simulink model "quadrotor_model50"  (R2021a)
settings: Solver=VariableStepAuto  StartTime=0.0  StopTime=40  RelTol=1e-1
values from neighbouring files (symbols this model uses):
  X = [X realx(index)]    [Plot_drone_3D.m]    (also in Plot_drone_3D_sub.m)
  Y = [Y realy(index)]    [Plot_drone_3D.m]    (also in Plot_drone_3D_sub.m)
  Z = [Z realz(index)]    [Plot_drone_3D.m]    (also in Plot_drone_3D_sub.m)
undefined symbols (not defined in the file or in its folder): Discrete, Time
libraries: sm_lib x6, sharedTrackingLibrary x4, sharedtransform x3, vrlib x2, aerolibutil x2, nesl_utility x1, dspmtrx3 x1, ctrlSharedLib x1
(part 2 of 2)

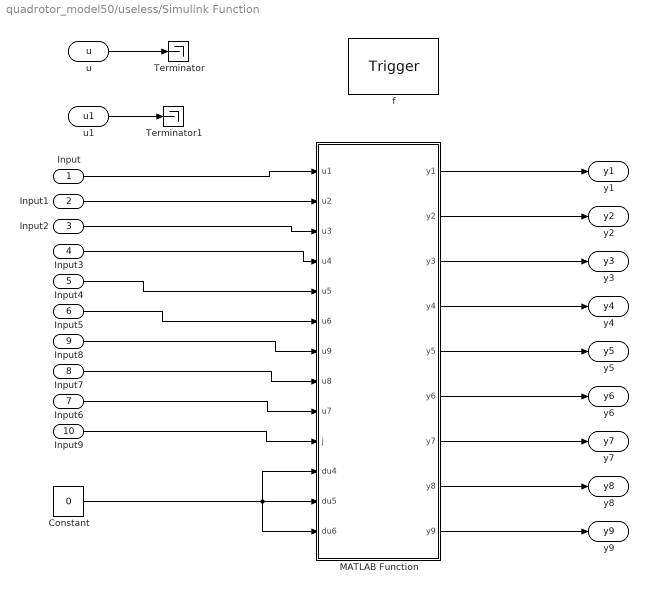
== system quadrotor_model50/useless/Simulink Function ==
  Input : Inport
  Input1 : Inport  Port=2
  Input2 : Inport  Port=3
  Input3 : Inport  Port=4
  Input4 : Inport  Port=5
  Input5 : Inport  Port=6
  Input6 : Inport  Port=7
  Input7 : Inport  Port=8
  Input8 : Inport  Port=9
  Input9 : Inport  Port=10
  f : TriggerPort  TriggerType=function-call  IsSimulinkFunction=on  FunctionName=suktee  FunctionVisibility=scoped  VariantControl=(inherit)
  Constant : Constant  Value=0
  MATLAB Function : MATLAB Function  TreatAsAtomicUnit=on
  Terminator : Terminator
  Terminator1 : Terminator
  u : ArgIn  DisableCoverage=on  ArgumentName=u
  u1 : ArgIn  DisableCoverage=on  Port=2  ArgumentName=u1
  y1 : ArgOut  DisableCoverage=on  ArgumentName=y1
  y2 : ArgOut  DisableCoverage=on  Port=2  ArgumentName=y2
  y3 : ArgOut  DisableCoverage=on  Port=3  ArgumentName=y3
  y4 : ArgOut  DisableCoverage=on  Port=4  ArgumentName=y4
  y5 : ArgOut  DisableCoverage=on  Port=5  ArgumentName=y5
  y6 : ArgOut  DisableCoverage=on  Port=6  ArgumentName=y6
  y7 : ArgOut  DisableCoverage=on  Port=7  ArgumentName=y7
  y8 : ArgOut  DisableCoverage=on  Port=8  ArgumentName=y8
  y9 : ArgOut  DisableCoverage=on  Port=9  ArgumentName=y9
  wires:
  Input/1 -> MATLAB Function/1(u1)
  Input1/1 -> MATLAB Function/2(u2)
  Input2/1 -> MATLAB Function/3(u3)
  Input4/1 -> MATLAB Function/5(u5)
  Input5/1 -> MATLAB Function/6(u6)
  Input7/1 -> MATLAB Function/8(u8)
  Input8/1 -> MATLAB Function/7(u9)
  Input6/1 -> MATLAB Function/9(u7)
  Input9/1 -> MATLAB Function/10(j)
  Input3/1 -> MATLAB Function/4(u4)
  MATLAB Function/1(y1) -> y1/1
  MATLAB Function/2(y2) -> y2/1
  MATLAB Function/3(y3) -> y3/1
  MATLAB Function/4(y4) -> y4/1
  MATLAB Function/5(y5) -> y5/1
  MATLAB Function/6(y6) -> y6/1
  MATLAB Function/9(y9) -> y9/1
  MATLAB Function/8(y8) -> y8/1
  MATLAB Function/7(y7) -> y7/1
  Constant/1 -> MATLAB Function/11(du4), MATLAB Function/13(du6), MATLAB Function/12(du5)
  u/1 -> Terminator/1
  u1/1 -> Terminator1/1

== system quadrotor_model50/useless/Simulink Function1 ==
  Input : Inport
  Input1 : Inport  Port=2
  Input2 : Inport  Port=3
  f : TriggerPort  TriggerType=function-call  IsSimulinkFunction=on  FunctionName=meas  FunctionVisibility=scoped  VariantControl=(inherit)
  y1 : ArgOut  DisableCoverage=on  ArgumentName=y1
  y2 : ArgOut  DisableCoverage=on  Port=2  ArgumentName=y2
  y3 : ArgOut  DisableCoverage=on  Port=3  ArgumentName=y3
  wires:
  Input/1 -> y1/1
  Input1/1 -> y2/1
  Input2/1 -> y3/1

== system quadrotor_model50/useless/Simulink Function2 ==
  jx : Inport
  jy : Inport  Port=2
  jz : Inport  Port=3
  jaba : TriggerPort  TriggerType=function-call  IsSimulinkFunction=on  FunctionName=jaba  FunctionVisibility=scoped  VariantControl=(inherit)
  MATLAB Function4 : MATLAB Function  TreatAsAtomicUnit=on
  y : ArgOut  DisableCoverage=on  ArgumentName=y
  wires:
  jy/1 -> MATLAB Function4/2(jy)
  jx/1 -> MATLAB Function4/1(jx)
  jz/1 -> MATLAB Function4/3(jz)
  MATLAB Function4/1(a) -> y/1

== system quadrotor_model50/useless/Simulink Function3 ==
  Input : Inport
  messi : TriggerPort  TriggerType=function-call  IsSimulinkFunction=on  FunctionName=messi  FunctionVisibility=scoped  VariantControl=(inherit)
  Demux : Demux  Outputs=3
  y : ArgOut  DisableCoverage=on  ArgumentName=y
  y1 : ArgOut  DisableCoverage=on  Port=2  ArgumentName=y1
  y2 : ArgOut  DisableCoverage=on  Port=3  ArgumentName=y2
  wires:
  Demux/3 -> y2/1
  Demux/1 -> y/1
  Demux/2 -> y1/1
  Input/1 -> Demux/1

== system quadrotor_model50/Quadrotor/Dynamics Model/Orientation Dynamics ==
  tau : Inport
  w : Inport  Port=2
  Body Inertia Matrix : Constant  Value=I
  Cross Product : vrlib/Utilities/Cross Product
  Matrix Multiply : Product  Multiplication=Matrix(*)
  Product : Product  Inputs=/*  Multiplication=Matrix(*)  OutDataTypeStr=Inherit: Inherit via back propagation
  Sum : Sum  Inputs=+-|
  dw : Outport
  wires:
  Body Inertia Matrix/1 -> Product/1, Matrix Multiply/1
  Matrix Multiply/1 -> Cross Product/2
  w/1 -> Cross Product/1, Matrix Multiply/2
  Cross Product/1 -> Sum/2
  tau/1 -> Sum/1
  Sum/1 -> Product/2
  Product/1 -> dw/1

== system quadrotor_model50/Quadrotor/Dynamics Model/Position Dynamics ==
  f : Inport
  Mass : Constant  Value=m
  Product1 : Product  Inputs=*/
  dv : Outport
  wires:
  Product1/1 -> dv/1
  f/1 -> Product1/1
  Mass/1 -> Product1/2

== system quadrotor_model50/Quadrotor/KInematics Model /Orientation Kinematics ==
  w : Inport
  q : Inport  Port=2
  Cross Product : vrlib/Utilities/Cross Product
  Demux : Demux
  Dot Product : DotProduct  InputSameDT=on  OutDataTypeStr=Inherit: Inherit via internal rule
  Gain1 : Gain  Gain=-1
  Mux : Mux  Inputs=3
  Mux1 : Mux  Inputs=2
  Product : Product
  Sum : Sum  Inputs=|++
  dq : Outport
  wires:
  q/1 -> Demux/1  "q"
  Demux/2 -> Mux/1
  Demux/3 -> Mux/2
  w/1 -> Product/2, Dot Product/2, Cross Product/2  "w"
  Demux/4 -> Mux/3
  Mux/1 -> Dot Product/1, Cross Product/1  "q_v"
  Mux1/1 -> dq/1
  Demux/1 -> Product/1  "q_0"
  Product/1 -> Sum/1
  Cross Product/1 -> Sum/2
  Sum/1 -> Mux1/2
  Dot Product/1 -> Gain1/1
  Gain1/1 -> Mux1/1

== system quadrotor_model50/Quadrotor/KInematics Model /Position Kinematics ==
  v : Inport
  dp : Outport
  wires:
  v/1 -> dp/1

== system quadrotor_model50/Quadrotor/KInematics Model /Vector Normalization ==
  v : Inport
  Dot Product1 : DotProduct  InputSameDT=on  OutDataTypeStr=Inherit: Inherit via internal rule
  Product3 : Product  Inputs=*/
  Sqrt : Sqrt  SaturateOnIntegerOverflow=on
  v' : Outport
  wires:
  Product3/1 -> v'/1
  v/1 -> Dot Product1/2, Product3/1, Dot Product1/1
  Dot Product1/1 -> Sqrt/1
  Sqrt/1 -> Product3/2

== system quadrotor_model50/Quadrotor/quat2Rotm/Skew Operator ==
  v : Inport
  Constant : Constant  Value=0
  Demux1 : Demux  Outputs=3
  Demux2 : Demux  Outputs=3
  Gain1 : Gain  Gain=-1
  Matrix Concatenate : Concatenate  NumInputs=3  Mode=Multidimensional array  ConcatenateDimension=2
  Mux1 : Mux  Inputs=3
  Mux2 : Mux  Inputs=3
  Mux3 : Mux  Inputs=3
  S : Outport
  wires:
  Constant/1 -> Mux3/3, Mux2/2, Mux1/1
  Demux1/3 -> Mux1/2
  Matrix Concatenate/1 -> S/1
  Demux1/1 -> Mux2/3
  v/1 -> Demux1/1, Gain1/1  "v"
  Demux2/1 -> Mux3/2
  Mux3/1 -> Matrix Concatenate/3
  Gain1/1 -> Demux2/1
  Demux2/3 -> Mux2/1
  Mux1/1 -> Matrix Concatenate/1
  Demux2/2 -> Mux1/3
  Demux1/2 -> Mux3/1
  Mux2/1 -> Matrix Concatenate/2

== system quadrotor_model50/Subsystem1/Subsystem/c ==
  y : Inport  SampleTime=1/100
  In2 : Inport  Port=2
  In3 : Inport  Port=3
  Constant : Constant
  Constant1 : Constant  Value=0
  Cos : Trigonometry  Operator=cos
  Cos1 : Trigonometry  Operator=cos
  Divide : Product  Inputs=**
  Divide1 : Product  Inputs=*/
  MATLAB Function : MATLAB Function  TreatAsAtomicUnit=on
  Mux : Mux  Inputs=36
  Reshape : Reshape  OutputDimensionality=Customize  OutputDimensions=[4,9]
  c : Outport  SampleTime=1/100
  wires:
  In2/1 -> Cos/1
  In3/1 -> Cos1/1
  Cos/1 -> Divide/1
  Cos1/1 -> Divide/2
  Constant/1 -> Divide1/1
  Divide/1 -> Divide1/2
  y/1 -> MATLAB Function/1(u)
  Divide1/1 -> Mux/12
  MATLAB Function/1(r1) -> Mux/25
  MATLAB Function/2(r2) -> Mux/26
  MATLAB Function/3(r3) -> Mux/27
  MATLAB Function/4(r4) -> Mux/29
  MATLAB Function/5(r5) -> Mux/30
  MATLAB Function/6(r6) -> Mux/31
  MATLAB Function/7(r7) -> Mux/33
  MATLAB Function/8(r8) -> Mux/34
  MATLAB Function/9(r9) -> Mux/35
  Constant1/1 -> Mux/24, Mux/23, Mux/22, Mux/21, Mux/20, Mux/19, Mux/18, Mux/17, Mux/16, Mux/15, Mux/14, Mux/13, Mux/11, Mux/10, Mux/9, Mux/8, Mux/7, Mux/6, Mux/5, Mux/4, Mux/3, Mux/2, Mux/1, Mux/28, Mux/32, Mux/36
  Mux/1 -> Reshape/1
  Reshape/1 -> c/1

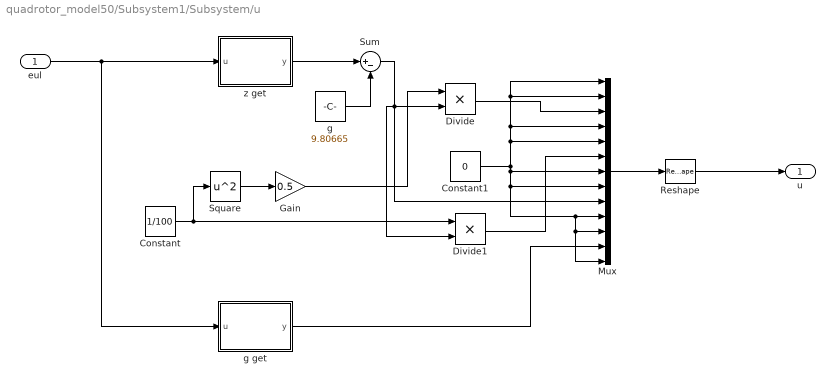
== system quadrotor_model50/Subsystem1/Subsystem/u ==
  eul : Inport
  Constant : Constant  Value=1/100
  Constant1 : Constant  Value=0
  Divide : Product  Inputs=**
  Divide1 : Product  Inputs=**
  Gain : Gain  Gain=0.5
  Mux : Mux  Inputs=13
  Reshape : Reshape  OutputDimensionality=Customize  OutputDimensions=[13,1]
  Square : Math  Operator=square  SaturateOnIntegerOverflow=on
  Sum : Sum  Inputs=|+-
  g : Constant  Value=9.80665
  g get : MATLAB Function  TreatAsAtomicUnit=on
  z get : MATLAB Function  TreatAsAtomicUnit=on
  u : Outport  SampleTime=1/100
  wires:
  Constant/1 -> Divide1/1, Square/1
  Square/1 -> Gain/1
  eul/1 -> g get/1(u), z get/1(u)
  z get/1(y) -> Sum/1
  g/1 -> Sum/2
  Gain/1 -> Divide/1
  Sum/1 -> Mux/9, Divide/2, Divide1/2
  Divide/1 -> Mux/3
  Divide1/1 -> Mux/6
  g get/1(y) -> Mux/12
  Constant1/1 -> Mux/13, Mux/11, Mux/10, Mux/8, Mux/7, Mux/5, Mux/4, Mux/1, Mux/2
  Mux/1 -> Reshape/1
  Reshape/1 -> u/1

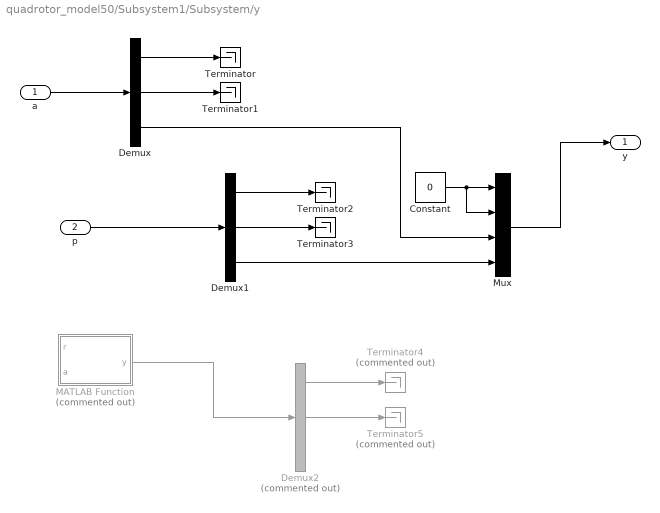
== system quadrotor_model50/Subsystem1/Subsystem/y ==
  a : Inport
  p : Inport  Port=2
  Constant : Constant  Value=0
  Demux : Demux  Outputs=3
  Demux1 : Demux  Outputs=3
  Demux2 : Demux  Commented=on  Outputs=3
  MATLAB Function : MATLAB Function  Commented=on  TreatAsAtomicUnit=on
  Mux : Mux
  Terminator{,1..3} (4 alike) : Terminator
  Terminator4 : Terminator  Commented=on
  Terminator5 : Terminator  Commented=on
  y : Outport  SampleTime=1/100
  wires:
  a/1 -> Demux/1
  Demux/1 -> Terminator/1
  Demux/2 -> Terminator1/1
  Demux1/2 -> Terminator3/1
  p/1 -> Demux1/1
  Demux1/1 -> Terminator2/1
  Demux1/3 -> Mux/4
  Constant/1 -> Mux/2, Mux/1
  Mux/1 -> y/1
  MATLAB Function/1(y) -> Demux2/1
  Demux2/2 -> Terminator5/1
  Demux2/1 -> Terminator4/1
  Demux/3 -> Mux/3

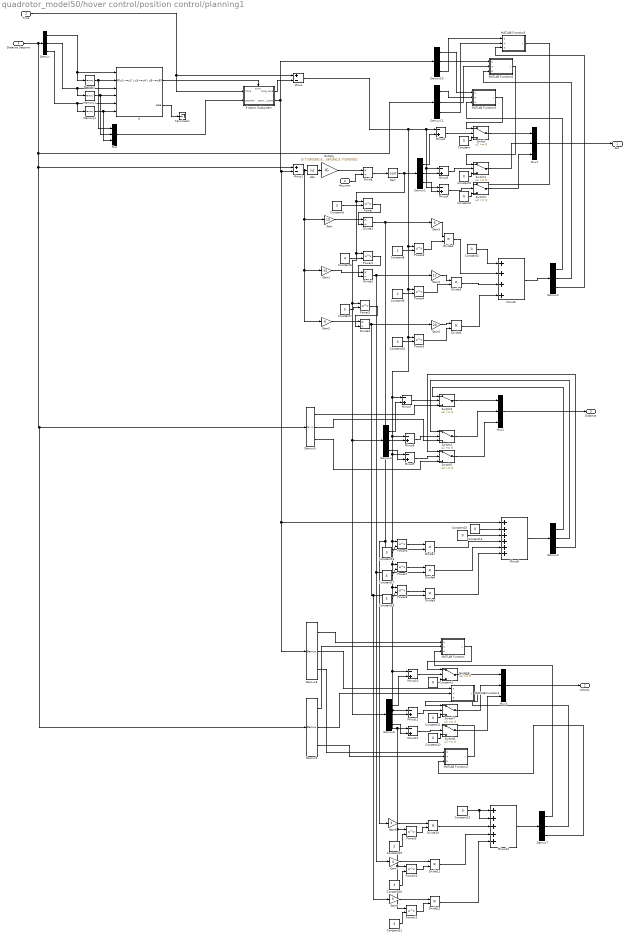
== system quadrotor_model50/hover control/position control/planning1 ==
  Distance Setpoint : Inport
  Time : Inport  Port=2
  Acc_max : Inport  Port=3
  Abs : Abs
  Constant{,1..4,11..15} (10 alike) : Constant  Value=0
  Constant{5,10,16,20} (4 alike) : Constant  Value=3
  Constant17 : Constant  Value=4
  Constant18 : Constant  Value=5
  Constant19 : Constant  Value=2
  Constant21 : Constant  Value=4
  Constant6 : Constant  Value=4
  Constant7 : Constant  Value=5
  Constant8 : Constant
  Constant9 : Constant  Value=2
  Demux{,1..11} (12 alike) : Demux  Outputs=3
  Divide{,1..3} (4 alike) : Product  Inputs=*/
  Divide{4..12} (9 alike) : Product  Inputs=**
  Gain : Gain  Gain=10
  Gain1 : Gain  Gain=-15
  Gain2 : Gain  Gain=6
  Gain3 : Gain  Gain=6
  Gain4 : Gain  Gain=12
  Gain5 : Gain  Gain=20
  Gain6 : Gain  Gain=3
  Gain7 : Gain  Gain=4
  Gain8 : Gain  Gain=5
  If : If  NumInputs=6  IfExpression=(u1~=u2 | u3~=u4 | u5~=u6)
  If Action Subsystem : Subsystem  TreatAsAtomicUnit=on
  MATLAB Function : MATLAB Function  TreatAsAtomicUnit=on
  MATLAB Function1 : MATLAB Function  TreatAsAtomicUnit=on
  MATLAB Function2 : MATLAB Function  TreatAsAtomicUnit=on
  MATLAB Function3 : MATLAB Function  TreatAsAtomicUnit=on
  MATLAB Function4 : MATLAB Function  TreatAsAtomicUnit=on
  MATLAB Function5 : MATLAB Function  TreatAsAtomicUnit=on
  Memory : Memory
  Memory1 : Memory
  Memory2 : Memory
  Minus : Sum  Inputs=+-
  Minus1 : Sum  Inputs=+-
  Minus{2..4,7..12} (9 alike) : Sum  Inputs=-+
  Minus13 : Sum  Inputs=+++++
  Minus5 : Sum  Inputs=++++
  Minus6 : Sum  Inputs=++++++
  Multiply : Gain  Gain=[5.773502692;5.773502692;5.773502692]
  Mux{,1..3} (4 alike) : Mux  Inputs=3
  Power{,1..11} (12 alike) : Math  Operator=pow  SaturateOnIntegerOverflow=on
  Sqrt : Sqrt  SaturateOnIntegerOverflow=on
  Switch{,1..8} (9 alike) : Switch
  Terminator : Terminator
  "Acc " : Outport
  velocity : Outport  Port=2
  Distance : Outport  Port=3
  wires:
  If/1 -> If Action Subsystem/Action
  Memory/1 -> Mux/1, If/2
  Time/1 -> Minus/1, If Action Subsystem/1(Time)
  Demux/1 -> Memory/1, If/1
  Memory1/1 -> Mux/2, If/4
  Memory2/1 -> Mux/3, If/6
  Demux/2 -> Memory1/1, If/3
  Demux/3 -> Memory2/1, If/5
  Mux/1 -> If Action Subsystem/2(position)
  Multiply/1 -> Divide/1
  Acc_max/1 -> Divide/2
  Divide/1 -> Sqrt/1
  Constant/1 -> Switch/3
  Mux1/1 -> "Acc "/1
  Switch/1 -> Mux1/1
  Constant3/1 -> Switch1/3
  Constant4/1 -> Switch2/3
  Switch1/1 -> Mux1/2
  Switch2/1 -> Mux1/3
  Demux1/2 -> Minus3/2
  Minus3/1 -> Switch1/2
  Demux1/3 -> Minus4/2
  Minus4/1 -> Switch2/2
  Gain/1 -> Divide1/1
  Constant5/1 -> Power/2
  Power/1 -> Divide1/2
  Constant6/1 -> Power1/2
  Gain1/1 -> Divide2/1
  Power1/1 -> Divide2/2
  Constant7/1 -> Power2/2
  Demux1/1 -> Minus2/2
  Minus1/1 -> Gain1/1, Gain2/1, Gain/1, Abs/1
  Power2/1 -> Divide3/2
  Gain2/1 -> Divide3/1
  Minus5/1 -> Demux2/1
  Demux2/1 -> MATLAB Function3/3(e)
  Demux2/3 -> MATLAB Function5/3(e)
  Constant2/1 -> Minus5/1
  Gain3/1 -> Divide4/1
  Divide4/1 -> Minus5/2
  Gain4/1 -> Divide5/1
  Divide5/1 -> Minus5/3
  Gain5/1 -> Divide6/1
  Divide6/1 -> Minus5/4
  Power3/1 -> Divide4/2
  Constant8/1 -> Power3/2
  Constant9/1 -> Power4/2
  Constant10/1 -> Power5/2
  Minus2/1 -> Switch/2
  Power4/1 -> Divide5/2
  Power5/1 -> Divide6/2
  Switch5/1 -> Mux2/3
  Minus7/1 -> Switch3/2
  Demux4/1 -> Minus7/2
  Demux4/3 -> Minus9/2
  Demux3/3 -> Switch5/1
  Switch3/1 -> Mux2/1
  Demux3/2 -> Switch4/1
  Demux3/1 -> Switch3/1
  Minus9/1 -> Switch5/2
  Minus8/1 -> Switch4/2
  Demux4/2 -> Minus8/2
  Switch4/1 -> Mux2/2
  Demux5/3 -> Switch5/3
  Demux5/1 -> Switch3/3
  Demux5/2 -> Switch4/3
  Mux2/1 -> Distance/1
  Minus6/1 -> Demux3/1
  If Action Subsystem/2(position_save) -> Demux8/1, Minus6/1, Minus1/2, Demux10/1
  Constant14/1 -> Minus6/2
  Constant15/1 -> Minus6/3
  Divide7/1 -> Minus6/4
  Divide8/1 -> Minus6/5
  Divide9/1 -> Minus6/6
  Power6/1 -> Divide7/1
  Power7/1 -> Divide8/1
  Power8/1 -> Divide9/1
  Constant16/1 -> Power6/2
  Constant17/1 -> Power7/2
  Constant18/1 -> Power8/2
  Distance Setpoint/1 -> Demux9/1, Demux5/1, Minus1/1, Demux11/1, Demux/1
  Abs/1 -> Multiply/1
  Switch8/1 -> Mux3/3
  Minus10/1 -> Switch6/2
  Sqrt/1 -> Demux4/1, Demux6/1, Power2/1, Power1/1, Power/1, Demux1/1
  Demux6/1 -> Minus10/2
  Demux6/3 -> Minus12/2
  Demux7/3 -> MATLAB Function2/3(e)
  Switch6/1 -> Mux3/1
  Demux7/2 -> MATLAB Function1/3(e)
  Demux7/1 -> MATLAB Function/3(e)
  Minus/1 -> Minus4/1, Minus3/1, Minus2/1, Power3/1, Minus7/1, Power6/1, Minus10/1, Minus11/1, Power9/1, Power11/1, Power10/1, Minus12/1, Power8/1, Power7/1, Minus9/1, Minus8/1, Power5/1, Power4/1
  Minus12/1 -> Switch8/2
  Minus11/1 -> Switch7/2
  Demux6/2 -> Minus11/2
  Switch7/1 -> Mux3/2
  Constant12/1 -> Switch8/3
  Constant1/1 -> Switch6/3
  Constant11/1 -> Switch7/3
  Mux3/1 -> velocity/1
  Minus13/1 -> Demux7/1
  Constant13/1 -> Minus13/2, Minus13/1
  Divide10/1 -> Minus13/3
  Divide11/1 -> Minus13/4
  Divide12/1 -> Minus13/5
  Gain6/1 -> Divide10/1
  Gain7/1 -> Divide11/1
  Gain8/1 -> Divide12/1
  Divide1/1 -> Gain3/1, Gain6/1, Divide7/2
  Divide2/1 -> Gain4/1, Gain7/1, Divide8/2
  Divide3/1 -> Gain5/1, Gain8/1, Divide9/2
  Power9/1 -> Divide10/2
  Power11/1 -> Divide12/2
  Power10/1 -> Divide11/2
  Constant19/1 -> Power9/2
  Constant20/1 -> Power10/2
  Constant21/1 -> Power11/2
  Demux8/1 -> MATLAB Function/1(q)
  Demux9/1 -> MATLAB Function/2(w)
  MATLAB Function/1(y) -> Switch6/1
  Demux8/2 -> MATLAB Function1/1(q)
  Demux9/2 -> MATLAB Function1/2(w)
  MATLAB Function1/1(y) -> Switch7/1
  Demux8/3 -> MATLAB Function2/1(q)
  Demux9/3 -> MATLAB Function2/2(w)
  MATLAB Function2/1(y) -> Switch8/1
  Demux10/1 -> MATLAB Function3/1(q)
  Demux11/1 -> MATLAB Function3/2(w)
  Demux10/2 -> MATLAB Function4/1(q)
  Demux11/2 -> MATLAB Function4/2(w)
  Demux2/2 -> MATLAB Function4/3(e)
  MATLAB Function4/1(y) -> Switch1/1
  Demux11/3 -> MATLAB Function5/2(w)
  Demux10/3 -> MATLAB Function5/1(q)
  MATLAB Function5/1(y) -> Switch2/1
  If Action Subsystem/1("time_save ") -> Minus/2
  MATLAB Function3/1(y) -> Switch/1
  If/2 -> Terminator/1

== system quadrotor_model50/hover control/position control/planning1/If Action Subsystem ==
  Time : Inport
  position : Inport  Port=2
  Action Port : ActionPort  InitializeStates=reset  PropagateVarSize=During execution  ActionPortLabel=if((u1~=u2 | u3~=u4 | u5~=u6))
  "time_save " : Outport
  position_save : Outport  Port=2
  wires:
  Time/1 -> "time_save "/1
  position/1 -> position_save/1

== matlab function quadrotor_model50/Subsystem1/Subsystem/u/g get ==
  data: u input; y output
function y = fcn(u)
u = u*[0 0 -9.80665]'
y = u(3);

== matlab function quadrotor_model50/magnetometer/MATLAB Function ==
  data: u input; y output
function y = magnetometer(u)
% y = roty(u(2))*rotx(u(1))*rotz(u(3));
y = eul2rotm(u');

== matlab function quadrotor_model50/useless/MATLAB Function ==
  data: u input; j input; y1 output; du4 input; du5 input; du6 input; y2 output; y3 output; y4 output; y5 output; y6 output; y7 output; y8 output; y9 output
function [y1,y2,y3,y4,y5,y6,y7,y8,y9] = stateqqqq(u,j,du4,du5,du6)
dt = 0.01;
yy=j(2);
xx= j(3);
u1=u(1);u2=u(2);u3=u(3);u4=u(4);u5=u(5);u6=u(6);u7=u(9);u8=u(8);u9=u(7);


jr = [1 sin(xx)*tan(yy) cos(xx)*tan(yy);0 cos(xx) -sin(xx);0 sin(xx)/cos(yy) cos(xx)/cos(yy)];


q7 = u1*dt + u4*dt^2 + 0.5*du4*dt^3;
jx = jr*[1;0;0];
jx =jx(1);

q8 = u2*dt + u5*dt^2 + 0.5*du5*dt^3;
jy = jr*[0;1;0];
jy =jy(2);

q9 = u3*dt + u6*dt^2 + 0.5*du6*dt^3;
jz = jr*[0;0;1];
jz =jz(3);

y1 = u1 + u4*dt + 0.5*du4*dt^2;
y2 = u2 + u5*dt  + 0.5*du5*dt^2;
y3 = u3 + u6*dt  + 0.5*du6*dt^2;
y4 = u4 + du4*dt;
y5 = u5 + du5*dt;
y6 = u6 + du6*dt;
y7 = u7 + jx *q7;
y8 = u8 + jy *q8;
y9 = u9 + jz *q9;

== matlab function quadrotor_model50/useless/MATLAB Function1 ==
  data: u input; wx output; wy output; wz output; ax output; ay output; az output; rz output; ry output; rx output
function [wx,wy,wz,ax,ay,az,rz,ry,rx] = fcn(u)
wx=u(1);
wy=u(2);
wz=u(3);
ax=u(4);
ay=u(5);
az=u(6);
rz=u(7);
ry=u(8);
rx=u(9);

== matlab function quadrotor_model50/useless/MATLAB Function3 ==
  data: u input; wx output; wy output; wz output; ax output; ay output; az output; rz output; ry output; rx output
function [wx,wy,wz,ax,ay,az,rz,ry,rx] = fcn(u)
wx=u(1);
wy=u(2);
wz=u(3);
ax=u(4);
ay=u(5);
az=u(6);
rz=u(7);
ry=u(8);
rx=u(9);

== matlab function quadrotor_model50/hover control/position control/planning1/MATLAB Function ==
  data: q input; y output; w input; e input
function y = fcn(q,w,e)
  if(q==w)
    y=0;
  else 
    y = e; 
  end

end

== matlab function quadrotor_model50/hover control/position control/planning1/MATLAB Function1 ==
  data: q input; y output; w input; e input
function y = fcn(q,w,e)
  if(q==w)
    y=0;
  else 
    y = e; 
  end

end

== matlab function quadrotor_model50/hover control/position control/planning1/MATLAB Function2 ==
  data: q input; y output; w input; e input
function y = fcn(q,w,e)
  if(q==w)
    y=0;
  else 
    y = e; 
  end

end

== matlab function quadrotor_model50/hover control/position control/planning1/MATLAB Function3 ==
  data: q input; y output; w input; e input
function y = fcn(q,w,e)
  if(q==w)
    y=0;
  else 
    y = e; 
  end

end

== matlab function quadrotor_model50/hover control/position control/planning1/MATLAB Function4 ==
  data: q input; y output; w input; e input
function y = fcn(q,w,e)
  if(q==w)
    y=0;
  else 
    y = e; 
  end

end

== matlab function quadrotor_model50/hover control/position control/planning1/MATLAB Function5 ==
  data: q input; y output; w input; e input
function y = fcn(q,w,e)
  if(q==w)
    y=0;
  else 
    y = e; 
  end

end

== matlab function quadrotor_model50/useless/MATLAB Function4 ==
  data: j input; a output
function a = jabco(j)
jx = j*[1;0;0];
u4 =jx(1);

jy = j*[0;1;0];
u5 =jy(2);

jz = j*[0;0;1];
u6 = jz(3);

dt = 1/100;
a = [1 0 0 dt 0 0 0 0 0;0 1 0 0 dt 0 0 0 0;0 0 1 0 0 dt 0 0 0;0 0 0 1 0 0 0 0 0;0 0 0 0 1 0 0 0 0;0 0 0 0 0 1 0 0 0;u4*dt 0 0 u4*dt^2 0 0 1 0 0;0 u5*dt 0 0 u5*dt^2 0 0 1 0;0 0 u6*dt 0 0 u6*dt^2 0 0 1];

== matlab function quadrotor_model50/useless/euler rate1 ==
  data: u input; j output
function j = fcn(u)
%z= u(1);
y=u(2);
x= u(3);

j = [1 sin(x)*tan(y) cos(x)*tan(y);0 cos(x) -sin(x);0 sin(x)/cos(y) cos(x)/cos(y)]

== matlab function quadrotor_model50/useless/Simulink Function/MATLAB Function ==
  data: u1 input; u2 input; u3 input; u4 input; u5 input; u6 input; u9 input; u8 input; u7 input; j input; y1 output; du4 input; du5 input; du6 input; y2 output; y3 output; y4 output; y5 output; y6 output; y7 output; y8 output; y9 output
function [y1,y2,y3,y4,y5,y6,y7,y8,y9] = stateqqqq(u1,u2,u3,u4,u5,u6,u9,u8,u7,j,du4,du5,du6)
dt = 0.01;
%yy=j(2);
%xx= j(3);
%u1=u(1);u2=u(2);u3=u(3);u4=u(4);u5=u(5);u6=u(6);u7=u(9);u8=u(8);u9=u(7);


%jr = [1 sin(xx)*tan(yy) cos(xx)*tan(yy);0 cos(xx) -sin(xx);0 sin(xx)/cos(yy) cos(xx)/cos(yy)];


q9 = u1*dt + u4*dt^2 + 0.5*du4*dt^3;
jx = j*[1;0;0];
jx =jx(1);

q8 = u2*dt + u5*dt^2 + 0.5*du5*dt^3;
jy = j*[0;1;0];
jy =jy(2);

q7 = u3*dt + u6*dt^2 + 0.5*du6*dt^3;
jz = j*[0;0;1];
jz =jz(3);

y1 = abs(u1 + u4*dt + 0.5*du4*dt^2);
y2 = abs(u2 + u5*dt  + 0.5*du5*dt^2);
y3 = abs(u3 + u6*dt  + 0.5*du6*dt^2);
y4 = abs(u4 + du4*dt);
y5 = abs(u5 + du5*dt);
y6 = abs(u6 + du6*dt);
y7 = abs(u7 + jx *q7);
y8 = abs(u8 + jy *q8);
y9 = abs(u9 + jz *q9);

== matlab function quadrotor_model50/useless/Simulink Function2/MATLAB Function4 ==
  data: jx input; a output; jy input; jz input
function a = jabco(jx,jy,jz)

dt = 1/100;
a = [1 0 0 dt 0 0 0 0 0;0 1 0 0 dt 0 0 0 0;0 0 1 0 0 dt 0 0 0;0 0 0 1 0 0 0 0 0;0 0 0 0 1 0 0 0 0;0 0 0 0 0 1 0 0 0;jx*dt 0 0 jx*dt^2 0 0 1 0 0;0 jy*dt 0 0 jy*dt^2 0 0 1 0;0 0 jz*dt 0 0 jz*dt^2 0 0 1];

== matlab function quadrotor_model50/useless/euler rate2 ==
  data: u input; j output
function j = fcn(u)
%z= u(1);
y=u(2);
x= u(3);

j = [1 sin(x)*tan(y) cos(x)*tan(y);0 cos(x) -sin(x);0 sin(x)/cos(y) cos(x)/cos(y)]

== matlab function quadrotor_model50/Ultrasonic sensor/MATLAB Function ==
  data: u1 input; y output; u2 input
function y = measurement_pz(u1,u2)
y=cos(u1)*cos(u2);

== matlab function quadrotor_model50/Subsystem1/Subsystem/y/MATLAB Function ==
  data: r input; y output; a input
function y = fcn(r,a)
q=eul2rotm(r);

y = q*(a-[0;0;9.81]);

== matlab function quadrotor_model50/hover control/position control/MATLAB Function ==
  data: u input; y output
function y = checkNan(u)
if isnan(u(1))
    u(1) = 0;
end
if isnan(u(2))
    u(2) = 0;
end
if isnan(u(3))
    u(3) = 0;
end
        
y = u;

== matlab function quadrotor_model50/Quadrotor/MATLAB Function ==
  data: u input; y output
function y = quat2Rom(u)

y = quat2rotm(u');

== matlab function quadrotor_model50/hover control/Desire Angle/MATLAB Function2 ==
  data: u input; y output
function y = checkNan(u)
if isnan(u(1)) || isinf(u(1))
    u(1) = 0;
end
if isnan(u(2)) || isinf(u(2))
    u(2) = 0;
end
if isnan(u(3)) || isinf(u(3))
    u(3) = 0;
end
        
y = u;

== matlab function quadrotor_model50/Quadrotor/quat2Rotm2/MATLAB Function ==
  data: u input; y output
function y = skewOperator(u)

y =[0 -u(3) u(2) ; u(3) 0 -u(1) ; -u(2) u(1) 0 ];

== matlab function quadrotor_model50/hover control/MATLAB Function ==
  data: u input; y output
function y = checkNan(u)
if isnan(u(1))
    u(1) = 0;
end
if isnan(u(2))
    u(2) = 0;
end
if isnan(u(3))
    u(3) = 0;
end
        
y = u;

== matlab function quadrotor_model50/Subsystem1/Subsystem/euler ==
  data: u input; y output
function y  = fcn(u)

y = eul2rotm(u);

== matlab function quadrotor_model50/Subsystem1/Subsystem/u/z get ==
  data: u input; y output
function y = fcn(u)
 u = u*[0 0 1]'
y = u(3);

== matlab function quadrotor_model50/Subsystem1/Subsystem/c/MATLAB Function ==
  data: u input; r1 output; r2 output; r3 output; r4 output; r5 output; r6 output; r7 output; r8 output; r9 output
function [r1,r2,r3,r4,r5,r6,r7,r8,r9] = fcn(u)
 r1 = u(1,1)  
 r2 = u(1,2)
 r3 = u(1,3)
 r4 = u(2,1)
 r5 = u(2,2) 
 r6 = u(2,3)
 r7 = u(3,1)
 r8 = u(3,2)
 r9 = u(3,3)
